simulink model "sg_eeg_20ch_rt"  (R2025a)
settings: Solver=FixedStepDiscrete  StartTime=0.0  StopTime=inf  FixedStep=0.001  RelTol=1e-3
libraries: slrealtimeiplib x1
settings Model: Creator=sr810  LastModifiedBy=sr810
settings SolverCC: ConcurrentTasks=on  PositivePriorityOrder=on
settings OptimizationCC: BlockReduction=off  OptimizeBlockIOStorage=off
settings DebuggingCC: TasksWithSamePriorityMsg=none
settings HardwareCC: ProdBitPerLong=64.0  ProdLongLongMode=on  ProdHWDeviceType=Intel->x86-64 (Linux 64)
settings RTWCC: SystemTargetFile=slrealtime.tlc  TemplateMakefile=slrealtime_default_tmf  Toolchain=Simulink Real-Time Toolchain  BuildConfiguration=Faster Runs  CodeExecutionProfiling=on  TargetLang=C++  Description=Simulink Real-Time
settings SimulinkRealTimeTargetCC: SLRTFileLogMaxRuns=1.0  ExtModeMaxTrigDuration=10.0  ExtModeStaticAllocSize=1000000.0  ExtModeTransport=0.0  MultiwordLength=2048.0  DynamicStringBufferSize=256.0  PreserveMATLABNamespacesInGeneratedCode=on  SubcomponentCodeInterfacePackaging=Reusable function  MATLABClassNameForMDSCustomization=Simulink.SoftwareTarget.GRTCustomization  InstructionSetFMA=off  LogToMDFFile=off

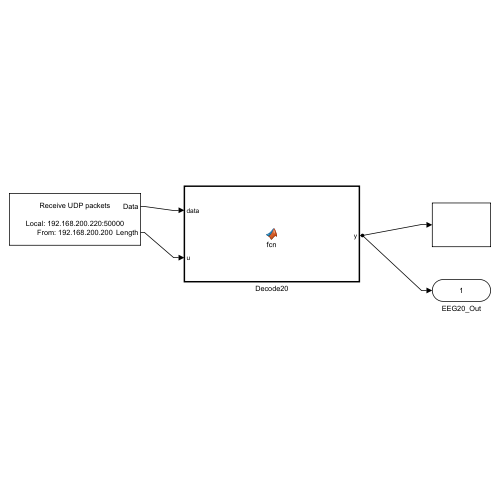
[thumbnail: Simulink's stored preview of the top-level diagram]
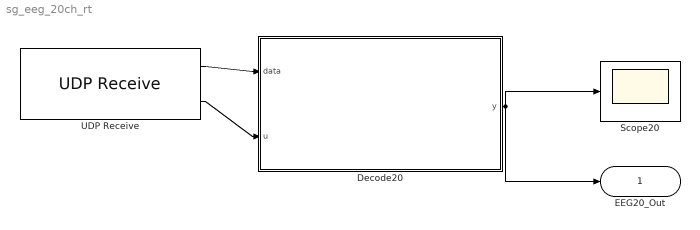
== system sg_eeg_20ch_rt ==
  Decode20 : MATLAB Function  TreatAsAtomicUnit=on
  Scope20 : Scope
  UDP Receive : slrealtimeiplib/UDP Receive  useHostTargetConn=off  ipAddress=192.168.200.220  localPort=50000  rcvWidth=1228  rcvFmAny=off  fmAddress=192.168.200.200  sampleTime=0.001  enableMessage=off  maxPackets=1
  EEG20_Out : Outport
  wires:
  UDP Receive/1 -> Decode20/1(data)
  UDP Receive/2 -> Decode20/2(u)
  Decode20/1(y) -> Scope20/1, EEG20_Out/1

== matlab function sg_eeg_20ch_rt/Decode20 ==
  data: data input; u input; y output
function y = fcn(data,u)
%#codegen
numChannels = 20;
y = zeros(numChannels,1);

nbytes = int32(u);
if nbytes < int32(28 + 3*numChannels)
    return;
end

payloadBytes = nbytes - int32(28);
bundleBytes = int32(3*numChannels);
if mod(payloadBytes, bundleBytes) ~= 0
    return;
end

numBundles = payloadBytes / bundleBytes;
startIdx = int32(29) + bundleBytes * (numBundles - int32(1));
if startIdx + bundleBytes - int32(1) > int32(numel(data))
    return;
end

for chn = 1:numChannels
    idx = double(startIdx + int32((chn-1)*3));
    b1 = uint32(data(idx));
    b2 = uint32(data(idx+1));
    b3 = uint32(data(idx+2));
    u24 = bitshift(b1,16) + bitshift(b2,8) + b3;
    if u24 >= uint32(2^23)
        s = int32(u24 - uint32(2^24));
    else
        s = int32(u24);
    end
    y(chn) = double(s);
end
